simulink model "mod5_Counter"  (R2020b)
settings: Solver=VariableStepAuto  StartTime=0.0  StopTime=inf  RelTol=1e-3
settings Model: EnablePacing=on  Creator=vigne  LastModifiedBy=sayali

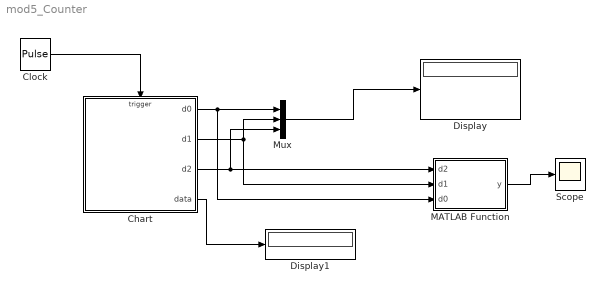
== system mod5_Counter ==
  Chart : Stateflow chart  TreatAsAtomicUnit=on
  Clock : DiscretePulseGenerator  PulseType=Time based  Period=0.5  PulseWidth=5
  Display : Display
  Display1 : Display
  MATLAB Function : MATLAB Function  TreatAsAtomicUnit=on
  Mux : Mux  Inputs=3
  Scope : Scope
  wires:
  Mux/1 -> Display/1
  Chart/1(d0) -> Mux/1, MATLAB Function/3(d0)
  Chart/2(d1) -> Mux/2, MATLAB Function/2(d1)
  Chart/3(d2) -> MATLAB Function/1(d2), Mux/3
  MATLAB Function/1(y) -> Scope/1
  Clock/1 -> Chart/Trigger
  Chart/4(data) -> Display1/1

== matlab function mod5_Counter/MATLAB Function ==
  data: d2 input; y output; d1 input; d0 input
function y= fcn(d2,d1,d0)
if(d2==0 && d1==0 && d0==0)
    y=0;
elseif(d2==0 && d1==0 && d0==1)
    y=1;
elseif(d2==0 && d1==1 && d0==0)
    y=2;
elseif(d2==0 && d1==1 && d0==1)
    y=3;
elseif(d2==1 && d1==0 && d0==0)
    y=4;
else
    y=0;
    
end

== stateflow chart mod5_Counter/Chart ==
  state digit0 [parallel]
    settings: executionOrder=1
    state zero
      en:
      d0=0;
    state one
      en:
      d0=1
    digit0.one -> digit0.zero [order 2] : [r==1]
    (default) -> digit0.zero
    digit0.one -> digit0.zero [order 1] : pulse{send(inc1);}
    digit0.zero -> digit0.one : pulse
  state check(d02,d01,d00) [function]
    (default) -> (junction 242) : % Conversion to Decimal
    (junction 242) -> (junction 236) [order 1] : [d02==0 && d01==0 && d00==0]
    (junction 242) -> (junction 237) [order 2]
    (junction 236) -> (junction 249) : {data=0;
        | r=0;}
    (junction 237) -> (junction 238) [order 1] : [d02==0 && d01==0 && d00==1]
    (junction 237) -> (junction 244) [order 2]
    (junction 238) -> (junction 248) : {data=1;
        | r=0;}
    (junction 244) -> (junction 241) [order 1] : [d02==0 && d01==1 && d00==0]
    (junction 244) -> (junction 239) [order 2]
    (junction 241) -> (junction 247) : {data=2;
        | r=0;}
    (junction 239) -> (junction 240) [order 1] : [d02==0 && d01==1 && d00==1]
    (junction 239) -> (junction 250) [order 2]
    (junction 240) -> (junction 245) : {data=3;
        | r=0;}
    (junction 250) -> (junction 260) [order 1] : [d02==1 && d01==0 && d00==0]
    (junction 250) -> (junction 243) [order 2]
    (junction 260) -> (junction 246) : {data=4;
        | r=0;}
    (junction 246) -> (junction 243)
    (junction 245) -> (junction 246)
    (junction 247) -> (junction 245)
    (junction 248) -> (junction 247)
    (junction 249) -> (junction 248)
    (junction 243) -> (junction 251)
  state digit1 [parallel]
    settings: executionOrder=2
    state zero
      en:
      d1=0;
    state one
      en:
      d1=1;
    (default) -> digit1.zero
    digit1.one -> digit1.zero : inc1{send(inc2);}
    digit1.zero -> digit1.one : inc1
  state digit2 [parallel]
    settings: executionOrder=3
    state zero
      en:
      d2=0;
    state one
      en:
      d2=1;
    (default) -> digit2.zero
    digit2.one -> digit2.zero : inc2
    digit2.zero -> digit2.one : inc2
  state ConversionState [parallel]
    during:
    data2=d2;
    data1=d1;
    data0=d0;
    r=0;
    check(data2,data1,data0);
    settings: executionOrder=4
  (default) -> digit0
  data: d02 function_input; d01 function_input; d00 function_input; d0 output; d1 output; d2 output; data output; data0 local; data1 local; data2 local; r local; re local; i local
  events: pulse input RISING_EDGE_EVENT; inc1 local FUNCTION_CALL_EVENT; inc2 local FUNCTION_CALL_EVENT; reset local EITHER_EDGE_EVENT
